simulink model "MSDR_DH_DeplV1sim"  (R2019a)
settings: Solver=ode45  StartTime=0.0  StopTime=simtime  FixedStep=0.1  MaxStep=ts_max  RelTol=rel_tolerance
values from neighbouring files (symbols this model uses):
  a_f = 1E-5*depl_fuel_temp_coef(depl_index)    [MSDR_DH_DeplV1para.m]
  a_g = 1E-5*depl_grap_temp_coef(depl_index)    [MSDR_DH_DeplV1para.m]
  A_s = 1.2245    [MSDR_DH_DeplV1para.m]
  beta = depl_beta(depl_index,:)    [MSDR_DH_DeplV1para.m]
  beta_t = sum(beta)    [MSDR_DH_DeplV1para.m]
  Cp_f = depl_Cp_Fuel_coef*1.355616e-3    [MSDR_DH_DeplV1para.m]
  Cp_p = Cp_s_shx    [MSDR_DH_DeplV1para.m]
  Cp_s = Cp_s*1e-6    (= 3.588208e-09)    [MSDR_DH_DeplV1para.m]
  Cp_sc = 4761.392e-6    (= 0.004761392)    [MSDR_DH_DeplV1para.m]
  Cp_w = 456.056e-6    (= 0.000456056)    [MSDR_DH_DeplV1para.m]
  D_it = 0.0141478    [MSDR_DH_DeplV1para.m]
  D_ot = 0.015875    [MSDR_DH_DeplV1para.m]
  DHRS_TIME_K = 10    [MSDR_DH_DeplV1para.m]
  dHs_dPs = -0.042433622114357    (= -0.0424336221144)    [MSDR_DH_DeplV1para.m]
  Epsilon = 1E-3    (= 0.001)    [MSDR_DH_DeplV1para.m]
  Fiss_factor = 2.464783802008740e-03    (= 0.00246478380201)    [MSDR_DH_DeplV1para.m]
  gamma0 = 9.635981959409105e-01    (= 0.963598195941)    [MSDR_DH_DeplV1para.m]
  gamma1 = 3.560674858154914e-02    (= 0.0356067485815)    [MSDR_DH_DeplV1para.m]
  gamma2 = 7.950554775404400e-04    (= 0.00079505547754)    [MSDR_DH_DeplV1para.m]
  gamma_I = 5.1135e-2    (= 0.051135)    [MSDR_DH_DeplV1para.m]
  gamma_Pm = 1.08E-2    (= 0.0108)    [MSDR_DH_DeplV1para.m]
  gamma_Xe = 1.1628e-2    (= 0.011628)    [MSDR_DH_DeplV1para.m]
  h_pw = h_s_shx    [MSDR_DH_DeplV1para.m]
  h_wb = 13349.334646671E-6    (= 0.0133493346467)    [MSDR_DH_DeplV1para.m]
  h_ws = 5732.378387768E-6    (= 0.00573237838777)    [MSDR_DH_DeplV1para.m]
  h_wsc = 8385.005556375E-6    (= 0.00838500555638)    [MSDR_DH_DeplV1para.m]
  hA_fg = [h_fg*A_fg/2, h_fg*A_fg/2]    [MSDR_DH_DeplV1para.m]
  hA_p_phx1 = h_p_phx*A_p_phx    [MSDR_DH_DeplV1para.m]
  hA_p_phx2 = h_p_phx*A_p_phx    [MSDR_DH_DeplV1para.m]
  hA_p_phx3 = h_p_phx*A_p_phx    [MSDR_DH_DeplV1para.m]
  hA_p_phx4 = h_p_phx*A_p_phx    [MSDR_DH_DeplV1para.m]
  hA_p_phx5 = h_p_phx*A_p_phx    [MSDR_DH_DeplV1para.m]
  hA_p_phx6 = h_p_phx*A_p_phx    [MSDR_DH_DeplV1para.m]
  hA_p_shx1 = h_p_shx*A_p_shx    [MSDR_DH_DeplV1para.m]
  hA_p_shx2 = h_p_shx*A_p_shx    [MSDR_DH_DeplV1para.m]
  hA_p_shx3 = h_p_shx*A_p_shx    [MSDR_DH_DeplV1para.m]
  hA_p_shx4 = h_p_shx*A_p_shx    [MSDR_DH_DeplV1para.m]
  hA_p_shx5 = h_p_shx*A_p_shx    [MSDR_DH_DeplV1para.m]
  hA_p_shx6 = h_p_shx*A_p_shx    [MSDR_DH_DeplV1para.m]
  hA_s_phx1 = h_s_phx*A_s_phx    [MSDR_DH_DeplV1para.m]
  hA_s_phx2 = h_s_phx*A_s_phx    [MSDR_DH_DeplV1para.m]
  hA_s_phx3 = h_s_phx*A_s_phx    [MSDR_DH_DeplV1para.m]
  hA_s_phx4 = h_s_phx*A_s_phx    [MSDR_DH_DeplV1para.m]
  hA_s_phx5 = h_s_phx*A_s_phx    [MSDR_DH_DeplV1para.m]
  hA_s_phx6 = h_s_phx*A_s_phx    [MSDR_DH_DeplV1para.m]
  hA_s_shx1 = h_s_shx*A_s_shx    [MSDR_DH_DeplV1para.m]
  hA_s_shx2 = h_s_shx*A_s_shx    [MSDR_DH_DeplV1para.m]
  hA_s_shx3 = h_s_shx*A_s_shx    [MSDR_DH_DeplV1para.m]
  hA_s_shx4 = h_s_shx*A_s_shx    [MSDR_DH_DeplV1para.m]
  hA_s_shx5 = h_s_shx*A_s_shx    [MSDR_DH_DeplV1para.m]
  hA_s_shx6 = h_s_shx*A_s_shx    [MSDR_DH_DeplV1para.m]
  I_0 = gamma_I*Sig_f_msdr*phi_0/lam_I    [MSDR_DH_DeplV1para.m]
  Ifa = [0.25, 0.25]    [MSDR_DH_DeplV1para.m]
  Ifb = [0.25, 0.25]    [MSDR_DH_DeplV1para.m]
  Ig = [0.5, 0.5]    [MSDR_DH_DeplV1para.m]
  K_1 = 11.632248097704855    (= 11.6322480977)    [MSDR_DH_DeplV1para.m]
  K_4 = b(1)    [MSDR_DH_DeplV1para.m]
  K_5 = a(1)    [MSDR_DH_DeplV1para.m]
  K_b = 12.834854076292217    (= 12.8348540763)    [MSDR_DH_DeplV1para.m]
  K_pump = 1/5    (= 0.2)    [MSDR_DH_DeplV1para.m]
  K_sc = -17.615718797133468    (= -17.6157187971)    [MSDR_DH_DeplV1para.m]
  ka = [0.235, 0.235]    [MSDR_DH_DeplV1para.m]
  kb = [0.235, 0.235]    [MSDR_DH_DeplV1para.m]
  kga = [0.015, 0.015]    [MSDR_DH_DeplV1para.m]
  kgb = [0.015, 0.015]    [MSDR_DH_DeplV1para.m]
  L = 8.5344    [MSDR_DH_DeplV1para.m]
  L_b = 2.3645    [MSDR_DH_DeplV1para.m]
  L_s = 4.723    [MSDR_DH_DeplV1para.m]
  Lam = depl_Lam(depl_index)    [MSDR_DH_DeplV1para.m]
  lam = [1.240E-02, 3.05E-02, 1.11E-01, 3.01E-01, 1.140E+00, 3.014E+00]    [MSDR_DH_DeplV1para.m]
  lam_bubl = 2.0e-2    (= 0.02)    [MSDR_DH_DeplV1para.m]
  lam_I = 2.875e-5    (= 2.875e-05)    [MSDR_DH_DeplV1para.m]
  lam_Pm = log(2)/(2.21*24*3600)    [MSDR_DH_DeplV1para.m]
  lam_Xe = 2.0916e-5    (= 2.0916e-05)    [MSDR_DH_DeplV1para.m]
  lambda0 = 0.0945298    [MSDR_DH_DeplV1para.m]
  lambda1 = 0.00441957    [MSDR_DH_DeplV1para.m]
  lambda2 = 8.60979e-05    [MSDR_DH_DeplV1para.m]
  m_3m = W_3*2    (= 8618.207327)    [MSDR_DH_DeplV1para.m]
  m_f_t = total_mp_phx + core_fm + mp_phxm*3 + m_fm    [MSDR_DH_DeplV1para.m]
  m_fm = W_f*1    (= 4989.48)    [MSDR_DH_DeplV1para.m]
  M_stm = 0.018    [MSDR_DH_DeplV1para.m]
  mcp_fa = mfa*Cp_f    [MSDR_DH_DeplV1para.m]
  mcp_fb = mfb*Cp_f    [MSDR_DH_DeplV1para.m]
  mcp_g = mg*Cp_g    [MSDR_DH_DeplV1para.m]
  mcp_p_phx1 = Cp_p_phx*mp_phx1    [MSDR_DH_DeplV1para.m]
  mcp_p_phx2 = Cp_p_phx*mp_phx2    [MSDR_DH_DeplV1para.m]
  mcp_p_phx3 = Cp_p_phx*mp_phx3    [MSDR_DH_DeplV1para.m]
  mcp_p_phx4 = Cp_p_phx*mp_phx4    [MSDR_DH_DeplV1para.m]
  mcp_p_phx5 = Cp_p_phx*mp_phx5    [MSDR_DH_DeplV1para.m]
  mcp_p_phx6 = Cp_p_phx*mp_phx6    [MSDR_DH_DeplV1para.m]
  mcp_p_shx1 = Cp_p_shx*mp_shx1    [MSDR_DH_DeplV1para.m]
  mcp_p_shx2 = Cp_p_shx*mp_shx2    [MSDR_DH_DeplV1para.m]
  mcp_p_shx3 = Cp_p_shx*mp_shx3    [MSDR_DH_DeplV1para.m]
  mcp_p_shx4 = Cp_p_shx*mp_shx4    [MSDR_DH_DeplV1para.m]
  mcp_p_shx5 = Cp_p_shx*mp_shx5    [MSDR_DH_DeplV1para.m]
  mcp_p_shx6 = Cp_p_shx*mp_shx6    [MSDR_DH_DeplV1para.m]
  mcp_s_phx1 = Cp_s_phx*ms_phx1    [MSDR_DH_DeplV1para.m]
  mcp_s_phx2 = Cp_s_phx*ms_phx2    [MSDR_DH_DeplV1para.m]
  mcp_s_phx3 = Cp_s_phx*ms_phx3    [MSDR_DH_DeplV1para.m]
  mcp_s_phx4 = Cp_s_phx*ms_phx4    [MSDR_DH_DeplV1para.m]
  mcp_s_phx5 = Cp_s_phx*ms_phx5    [MSDR_DH_DeplV1para.m]
  mcp_s_phx6 = Cp_s_phx*ms_phx6    [MSDR_DH_DeplV1para.m]
  mcp_s_shx1 = Cp_s_shx*ms_shx1    [MSDR_DH_DeplV1para.m]
  mcp_s_shx2 = Cp_s_shx*ms_shx1    [MSDR_DH_DeplV1para.m]
  mcp_s_shx3 = Cp_s_shx*ms_shx1    [MSDR_DH_DeplV1para.m]
  mcp_s_shx4 = Cp_s_shx*ms_shx1    [MSDR_DH_DeplV1para.m]
  mcp_s_shx5 = Cp_s_shx*ms_shx1    [MSDR_DH_DeplV1para.m]
  mcp_s_shx6 = Cp_s_shx*ms_shx1    [MSDR_DH_DeplV1para.m]
  mcp_t_phx1 = Cp_t_phx*mt_phx1    [MSDR_DH_DeplV1para.m]
  mcp_t_phx2 = Cp_t_phx*mt_phx2    [MSDR_DH_DeplV1para.m]
  mcp_t_phx3 = Cp_t_phx*mt_phx3    [MSDR_DH_DeplV1para.m]
  mcp_t_phx4 = Cp_t_phx*mt_phx4    [MSDR_DH_DeplV1para.m]
  mcp_t_phx5 = Cp_t_phx*mt_phx5    [MSDR_DH_DeplV1para.m]
  mcp_t_phx6 = Cp_t_phx*mt_phx6    [MSDR_DH_DeplV1para.m]
  mcp_t_shx1 = Cp_t_phx*mt_shx1    [MSDR_DH_DeplV1para.m]
  mcp_t_shx2 = Cp_t_phx*mt_shx2    [MSDR_DH_DeplV1para.m]
  mcp_t_shx3 = Cp_t_phx*mt_shx3    [MSDR_DH_DeplV1para.m]
  mcp_t_shx4 = Cp_t_phx*mt_shx4    [MSDR_DH_DeplV1para.m]
  mcp_t_shx5 = Cp_t_phx*mt_shx5    [MSDR_DH_DeplV1para.m]
  mcp_t_shx6 = Cp_t_phx*mt_shx6    [MSDR_DH_DeplV1para.m]
  ... (+159 more)
undefined symbols (not defined in the file or in its folder): C0, DHRS_MODE, DHRS_Power, DHRS_time, ln, P, Trip_P1_pump, Trip_P2_pump, Trip_P3_pump, Trip_S1_pump, Trip_S2_pump, Trip_S3_pump, Trip_T1_pump, Trip_T2_pump, Trip_T3_pump, Trip_UHX
libraries: simulink x2
(part 1 of 4)
settings Model: Creator=viikr  LastModifiedBy=visura
settings SolverCC: SolverJacobianMethodControl=FullAnalytical  AlgebraicLoopSolver=LineSearch
settings DataIOCC: ReturnWorkspaceOutputs=off
settings DebuggingCC: PregeneratedLibrarySubsystemCodeDiagnostic=none  ArithmeticOperatorsInVariantConditions=warning
settings SFSimCC: SimUseLocalCustomCode=off
settings RTWCC: RTWUseLocalCustomCode=off

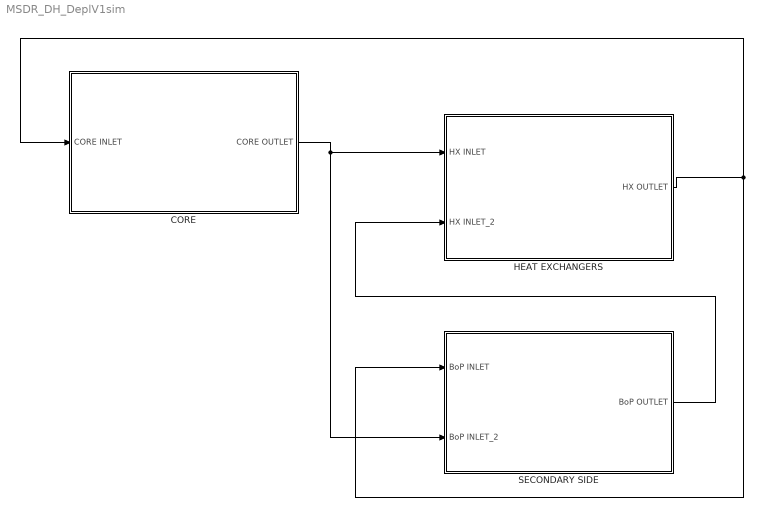
== system MSDR_DH_DeplV1sim ==
  CORE : Subsystem
  HEAT EXCHANGERS : Subsystem
  SECONDARY SIDE : Subsystem
  wires:
  SECONDARY SIDE/1(BoP OUTLET) -> HEAT EXCHANGERS/2(HX INLET_2)
  HEAT EXCHANGERS/1(HX OUTLET) -> SECONDARY SIDE/1(BoP INLET), CORE/1(CORE INLET)
  CORE/1(CORE OUTLET) -> SECONDARY SIDE/2(BoP INLET_2), HEAT EXCHANGERS/1(HX INLET)

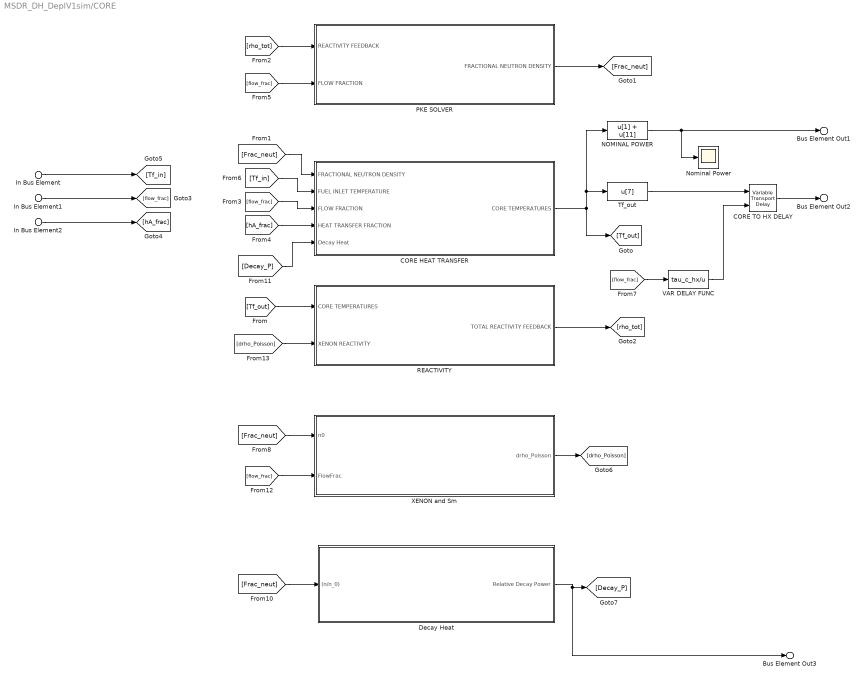
== system MSDR_DH_DeplV1sim/CORE ==
  In Bus Element2 : Inport  PortName=CORE INLET  Element=FUEL HEAT TRANSFER FRACTION
  In Bus Element : Inport  PortName=CORE INLET  Element=HX FUEL OUTLET TEMPERATURE
  In Bus Element1 : Inport  PortName=CORE INLET  Element=FUEL FLOW FRACTION
  CORE HEAT TRANSFER : Subsystem
  CORE TO HX DELAY : VariableTransportDelay  MaximumDelay=10000000  InitialOutput=T0_fb(2)
  Decay Heat : Subsystem
  NOMINAL POWER : Fcn  Expr=u[1] + u[11]
  Nominal Power : Scope
  PKE SOLVER : Subsystem
  REACTIVITY : Subsystem
  Tf_out : Fcn  Expr=u[7]
  VAR DELAY FUNC : Fcn  Expr=tau_c_hx/u
  XENON and Sm : Subsystem
  Bus Element Out2 : Outport  PortName=CORE OUTLET  Element=CORE FUEL OUTLET TEMPERATURE
  Bus Element Out1 : Outport  PortName=CORE OUTLET  Element=CORE POWER
  Bus Element Out3 : Outport  PortName=CORE OUTLET  Element=DECAY HEAT
  wires:
  Tf_out/1 -> CORE TO HX DELAY/1
  CORE HEAT TRANSFER/1(CORE TEMPERATURES) -> Tf_out/1, NOMINAL POWER/1, [Tf_out]
  [Tf_out] -> REACTIVITY/1(CORE TEMPERATURES)
  PKE SOLVER/1(FRACTIONAL NEUTRON DENSITY) -> [Frac_neut]
  [Frac_neut] -> CORE HEAT TRANSFER/1(FRACTIONAL NEUTRON DENSITY)
  REACTIVITY/1(TOTAL REACTIVITY FEEDBACK) -> [rho_tot]
  [flow_frac] -> PKE SOLVER/2(FLOW FRACTION)
  [flow_frac] -> CORE HEAT TRANSFER/3(FLOW FRACTION)
  [hA_frac] -> CORE HEAT TRANSFER/4(HEAT TRANSFER FRACTION)
  CORE TO HX DELAY/1 -> Bus Element Out2/1
  [flow_frac] -> VAR DELAY FUNC/1
  VAR DELAY FUNC/1 -> CORE TO HX DELAY/2
  [Tf_in] -> CORE HEAT TRANSFER/2(FUEL INLET TEMPERATURE)
  XENON and Sm/1(drho_Poisson) -> [drho_Poisson]
  [Frac_neut] -> XENON and Sm/1(n0)
  In Bus Element1/1 -> [flow_frac]
  In Bus Element2/1 -> [hA_frac]
  In Bus Element/1 -> [Tf_in]
  [drho_Poisson] -> REACTIVITY/2(XENON REACTIVITY)
  [rho_tot] -> PKE SOLVER/1(REACTIVITY FEEDBACK)
  [Frac_neut] -> Decay Heat/1((n/n_0))
  Decay Heat/1("Relative Decay Power ") -> Bus Element Out3/1, [Decay_P]
  [Decay_P] -> CORE HEAT TRANSFER/5(Decay Heat)
  NOMINAL POWER/1 -> Nominal Power/1, Bus Element Out1/1
  [flow_frac] -> XENON and Sm/2(FlowFrac)

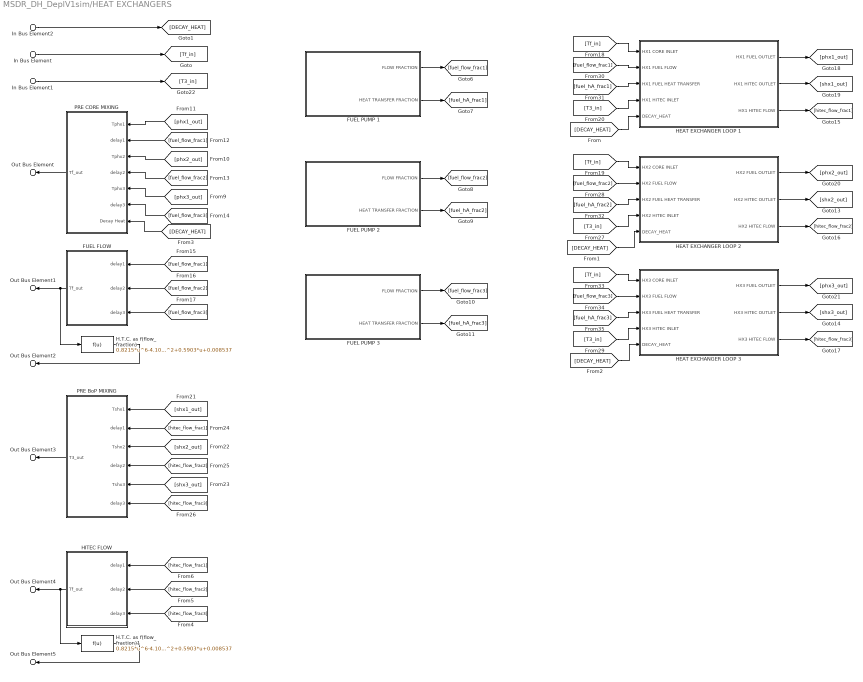
== system MSDR_DH_DeplV1sim/HEAT EXCHANGERS ==
  In Bus Element : Inport  PortName=HX INLET  Element=CORE FUEL OUTLET TEMPERATURE
  In Bus Element2 : Inport  PortName=HX INLET  Element=DECAY HEAT
  In Bus Element1 : Inport  Port=2  PortName=HX INLET_2  Element=BoP HITEC OUTLET TEMPERATURE
  FUEL FLOW : Subsystem
  FUEL PUMP 1 : Subsystem
  FUEL PUMP 2 : Subsystem
  FUEL PUMP 3 : Subsystem
  H.T.C. as f(flow_fraction) : Fcn  Expr=0.8215*u^6-4.108*u^5+7.848*u^4-7.165*u^3+3.004*u^2+0.5903*u+0.008537
  H.T.C. as f(flow_fraction)1 : Fcn  Expr=0.8215*u^6-4.108*u^5+7.848*u^4-7.165*u^3+3.004*u^2+0.5903*u+0.008537
  HEAT EXCHANGER LOOP 1 : Subsystem
  HEAT EXCHANGER LOOP 2 : Subsystem
  HEAT EXCHANGER LOOP 3 : Subsystem
  HITEC FLOW : Subsystem
  PRE BoP MIXING : Subsystem
  PRE CORE MIXING : Subsystem
  Out Bus Element : Outport  PortName=HX OUTLET  Element=HX FUEL OUTLET TEMPERATURE
  Out Bus Element1 : Outport  PortName=HX OUTLET  Element=FUEL FLOW FRACTION
  Out Bus Element2 : Outport  PortName=HX OUTLET  Element=FUEL HEAT TRANSFER FRACTION
  Out Bus Element3 : Outport  PortName=HX OUTLET  Element=HX HITEC OUTLET TEMPERATURE
  Out Bus Element4 : Outport  PortName=HX OUTLET  Element=HITEC FLOW FRACTION
  Out Bus Element5 : Outport  PortName=HX OUTLET  Element=HITEC HEAT TRANSFER FRACTION
  wires:
  In Bus Element/1 -> [Tf_in]
  FUEL PUMP 1/1(FLOW FRACTION) -> [fuel_flow_frac1]
  FUEL PUMP 1/2(HEAT TRANSFER FRACTION) -> [fuel_hA_frac1]
  FUEL PUMP 2/2(HEAT TRANSFER FRACTION) -> [fuel_hA_frac2]
  FUEL PUMP 2/1(FLOW FRACTION) -> [fuel_flow_frac2]
  FUEL PUMP 3/2(HEAT TRANSFER FRACTION) -> [fuel_hA_frac3]
  FUEL PUMP 3/1(FLOW FRACTION) -> [fuel_flow_frac3]
  [phx1_out] -> PRE CORE MIXING/1(Tphx1)
  [fuel_flow_frac1] -> PRE CORE MIXING/2(delay1)
  [phx2_out] -> PRE CORE MIXING/3(Tphx2)
  [fuel_flow_frac2] -> PRE CORE MIXING/4(delay2)
  [phx3_out] -> PRE CORE MIXING/5(Tphx3)
  [fuel_flow_frac3] -> PRE CORE MIXING/6(delay3)
  PRE CORE MIXING/1(Tf_out) -> Out Bus Element/1
  FUEL FLOW/1(Tf_out) -> H.T.C. as f(flow_fraction)/1, Out Bus Element1/1
  H.T.C. as f(flow_fraction)/1 -> Out Bus Element2/1
  [hitec_flow_frac2] -> PRE BoP MIXING/4(delay2)
  [hitec_flow_frac1] -> PRE BoP MIXING/2(delay1)
  [shx2_out] -> PRE BoP MIXING/3(Tshx2)
  [shx3_out] -> PRE BoP MIXING/5(Tshx3)
  [hitec_flow_frac3] -> PRE BoP MIXING/6(delay3)
  [shx1_out] -> PRE BoP MIXING/1(Tshx1)
  PRE BoP MIXING/1(T3_out) -> Out Bus Element3/1
  HEAT EXCHANGER LOOP 2/2(HX2 HITEC OUTLET) -> [shx2_out]
  [T3_in] -> HEAT EXCHANGER LOOP 3/4(HX3 HITEC INLET)
  HEAT EXCHANGER LOOP 3/3(HX3 HITEC FLOW) -> [hitec_flow_frac3]
  HEAT EXCHANGER LOOP 2/3(HX2 HITEC FLOW) -> [hitec_flow_frac2]
  HEAT EXCHANGER LOOP 1/3(HX1 HITEC FLOW) -> [hitec_flow_frac1]
  HEAT EXCHANGER LOOP 3/2(HX3 HITEC OUTLET) -> [shx3_out]
  HEAT EXCHANGER LOOP 1/2(HX1 HITEC OUTLET) -> [shx1_out]
  [T3_in] -> HEAT EXCHANGER LOOP 1/4(HX1 HITEC INLET)
  HEAT EXCHANGER LOOP 1/1(HX1 FUEL OUTLET) -> [phx1_out]
  [fuel_flow_frac3] -> HEAT EXCHANGER LOOP 3/2(HX3 FUEL FLOW)
  [Tf_in] -> HEAT EXCHANGER LOOP 2/1(HX2 CORE INLET)
  [T3_in] -> HEAT EXCHANGER LOOP 2/4(HX2 HITEC INLET)
  [fuel_hA_frac2] -> HEAT EXCHANGER LOOP 2/3(HX2 FUEL HEAT TRANSFER)
  [fuel_flow_frac2] -> HEAT EXCHANGER LOOP 2/2(HX2 FUEL FLOW)
  [Tf_in] -> HEAT EXCHANGER LOOP 3/1(HX3 CORE INLET)
  [fuel_hA_frac1] -> HEAT EXCHANGER LOOP 1/3(HX1 FUEL HEAT TRANSFER)
  [Tf_in] -> HEAT EXCHANGER LOOP 1/1(HX1 CORE INLET)
  [fuel_hA_frac3] -> HEAT EXCHANGER LOOP 3/3(HX3 FUEL HEAT TRANSFER)
  HEAT EXCHANGER LOOP 3/1(HX3 FUEL OUTLET) -> [phx3_out]
  HEAT EXCHANGER LOOP 2/1(HX2 FUEL OUTLET) -> [phx2_out]
  In Bus Element1/1 -> [T3_in]
  [fuel_flow_frac1] -> HEAT EXCHANGER LOOP 1/2(HX1 FUEL FLOW)
  [fuel_flow_frac1] -> FUEL FLOW/1(delay1)
  [fuel_flow_frac2] -> FUEL FLOW/2(delay2)
  [fuel_flow_frac3] -> FUEL FLOW/3(delay3)
  In Bus Element2/1 -> [DECAY_HEAT]
  [DECAY_HEAT] -> HEAT EXCHANGER LOOP 1/5(DECAY_HEAT)
  [DECAY_HEAT] -> HEAT EXCHANGER LOOP 2/5(DECAY_HEAT)
  [DECAY_HEAT] -> HEAT EXCHANGER LOOP 3/5(DECAY_HEAT)
  [DECAY_HEAT] -> PRE CORE MIXING/7(Decay Heat)
  [hitec_flow_frac1] -> HITEC FLOW/1(delay1)
  [hitec_flow_frac2] -> HITEC FLOW/2(delay2)
  [hitec_flow_frac3] -> HITEC FLOW/3(delay3)
  HITEC FLOW/1(Tf_out) -> H.T.C. as f(flow_fraction)1/1, Out Bus Element4/1
  H.T.C. as f(flow_fraction)1/1 -> Out Bus Element5/1

== system MSDR_DH_DeplV1sim/SECONDARY SIDE ==
  In Bus Element : Inport  PortName=BoP INLET  Element=HX HITEC OUTLET TEMPERATURE
  In Bus Element2 : Inport  PortName=BoP INLET  Element=HITEC FLOW FRACTION
  In Bus Element3 : Inport  PortName=BoP INLET  Element=HITEC HEAT TRANSFER FRACTION
  In Bus Element1 : Inport  Port=2  PortName=BoP INLET_2  Element=CORE POWER
  OTSG + BALANCE OF PLANT : Subsystem  Commented=on
  Variant Subsystem : Subsystem  Variant=on
  Bus Element Out2 : Outport  PortName=BoP OUTLET  Element=BoP HITEC OUTLET TEMPERATURE
  wires:
  Variant Subsystem/1(HITEC_OUTLET) -> Bus Element Out2/1
  In Bus Element3/1 -> Variant Subsystem/4(HITEC_HTC_FRAC)
  In Bus Element2/1 -> Variant Subsystem/3(HITEC_FLOW_FRAC)
  In Bus Element/1 -> Variant Subsystem/1(HITEC_INLET)
  In Bus Element1/1 -> Variant Subsystem/2(POWER LEVEL)

== system MSDR_DH_DeplV1sim/CORE/CORE HEAT TRANSFER ==
  FRACTIONAL NEUTRON DENSITY : Inport
  FUEL INLET TEMPERATURE : Inport  Port=2
  FLOW FRACTION : Inport  Port=3
  HEAT TRANSFER FRACTION : Inport  Port=4
  Decay Heat : Inport  Port=5
  Mux : Mux  Inputs=11
      settings: DisplayOption=signals
  T_f1a : Integrator  InitialCondition=T0_fa(1)
  T_f1b : Integrator  InitialCondition=T0_fb(1)
  T_f2a : Integrator  InitialCondition=T0_fa(2)
  T_f2b : Integrator  InitialCondition=T0_fb(2)
  T_g1 : Integrator  InitialCondition=T0_g(1)
  T_g2 : Integrator  InitialCondition=T0_g(2)
  To Workspace : ToWorkspace  VariableName=core_ht  SampleTime=-1
  d(T_f1a)/dt : Fcn  Expr=((u[9]*W_f/mfa(1))*(u[2] - u[3])) + (ka(1)*P*u[1]/mcp_fa(1)) + (kga(1)*u[10]*hA_fg(1)*(u[5] - u[3]))/((kga(1)+kgb(1))*mcp_fa(1)) + u(11)*P*mfa(1)/(m_f_t*mcp_fa(1))
  d(T_f1a)/dt1 : Fcn  Expr=(1-0.07)*u
  d(T_f1b)/dt : Fcn  Expr=((u[9]*W_f/mfb(1))*(u[3] - u[4])) + (kb(1)*P*u[1]/mcp_fb(1)) + (kgb(1)*u[10]*hA_fg(1)*(u[5] - u[3]))/((kga(1)+kgb(1))*mcp_fb(1)) + u(11)*P*mfb(1)/(m_f_t*mcp_fb(1))
  d(T_f2a)/dt : Fcn  Expr=((u[9]*W_f/mfa(2))*(u[4] - u[6])) + (ka(2)*P*u[1]/mcp_fa(2)) + (kga(2)*u[10]*hA_fg(2)*(u[8] - u[6]))/((kga(2)+kgb(2))*mcp_fa(2)) + u(11)*P*mfa(2)/(m_f_t*mcp_fa(2))
  d(T_f2b)/dt : Fcn  Expr=((u[9]*W_f/mfb(2))*(u[6] - u[7])) + (kb(2)*P*u[1]/mcp_fb(2)) + (kgb(2)*u[10]*hA_fg(2)*(u[8] - u[6]))/((kga(2)+kgb(2))*mcp_fb(2)) + u(11)*P*mfb(2)/(m_f_t*mcp_fb(2))
  d(T_g1)/dt : Fcn  Expr=(u[10]*hA_fg(1)/mcp_g(1))*(u[3] - u[5]) + (kga(1)+kgb(1))*P*u[1]/mcp_g(1)
  d(T_g2)/dt : Fcn  Expr=(u[10]*hA_fg(2)/mcp_g(2))*(u[6] - u[8]) + (kga(2)+kgb(2))*P*u[1]/mcp_g(2)
  CORE TEMPERATURES : Outport
  wires:
  d(T_f1b)/dt/1 -> T_f1b/1
  d(T_f1a)/dt/1 -> T_f1a/1
  d(T_g1)/dt/1 -> T_g1/1
  FUEL INLET TEMPERATURE/1 -> Mux/2
  T_f1a/1 -> Mux/3
  T_f1b/1 -> Mux/4
  T_g1/1 -> Mux/5
  d(T_f2a)/dt/1 -> T_f2a/1
  d(T_f2b)/dt/1 -> T_f2b/1
  T_g2/1 -> Mux/8
  d(T_g2)/dt/1 -> T_g2/1
  T_f2a/1 -> Mux/6
  T_f2b/1 -> Mux/7
  Mux/1 -> To Workspace/1, CORE TEMPERATURES/1, d(T_g2)/dt/1, d(T_f2b)/dt/1, d(T_f2a)/dt/1, d(T_g1)/dt/1, d(T_f1b)/dt/1, d(T_f1a)/dt/1
  FLOW FRACTION/1 -> Mux/9
  HEAT TRANSFER FRACTION/1 -> Mux/10
  Decay Heat/1 -> Mux/11
  d(T_f1a)/dt1/1 -> Mux/1
  FRACTIONAL NEUTRON DENSITY/1 -> d(T_f1a)/dt1/1

== system MSDR_DH_DeplV1sim/CORE/Decay Heat ==
  (n/n_0) : Inport
  Decay Power Percentage : Fcn  Expr=u(2)+u(3)+u(4)
  Decay Precursor G1 : Fcn  Expr=u(1)*Fiss_factor*gamma0 - lambda0*u(2)
  Decay Precursor G2 : Fcn  Expr=u(1)*Fiss_factor*gamma1 - lambda1*u(3)
  Decay Precursor G3 : Fcn  Expr=u(1)*Fiss_factor*gamma2 - lambda2*u(4)
  Integrator : Integrator  InitialCondition=0.025125
  Integrator1 : Integrator  InitialCondition=0.0198578
  Integrator2 : Integrator  InitialCondition=0.0227606
  Mux : Mux
      settings: DisplayOption=signals
  Scope : Scope
  To Workspace : ToWorkspace  VariableName=Decay_Group_total  SampleTime=-1
  To Workspace1 : ToWorkspace  VariableName=Decay_Groups1  SampleTime=-1
  To Workspace2 : ToWorkspace  VariableName=Decay_Groups2  SampleTime=-1
  To Workspace3 : ToWorkspace  VariableName=Decay_Groups3  SampleTime=-1
  "Relative Decay Power " : Outport
  wires:
  Decay Power Percentage/1 -> "Relative Decay Power "/1, Scope/1, To Workspace/1
  Decay Precursor G1/1 -> Integrator/1
  Decay Precursor G2/1 -> Integrator1/1
  Decay Precursor G3/1 -> Integrator2/1
  Mux/1 -> Decay Precursor G3/1, Decay Precursor G2/1, Decay Precursor G1/1, Decay Power Percentage/1
  Integrator/1 -> Mux/2, To Workspace1/1
  Integrator1/1 -> Mux/3, To Workspace2/1
  Integrator2/1 -> Mux/4, To Workspace3/1
  (n/n_0)/1 -> Mux/1

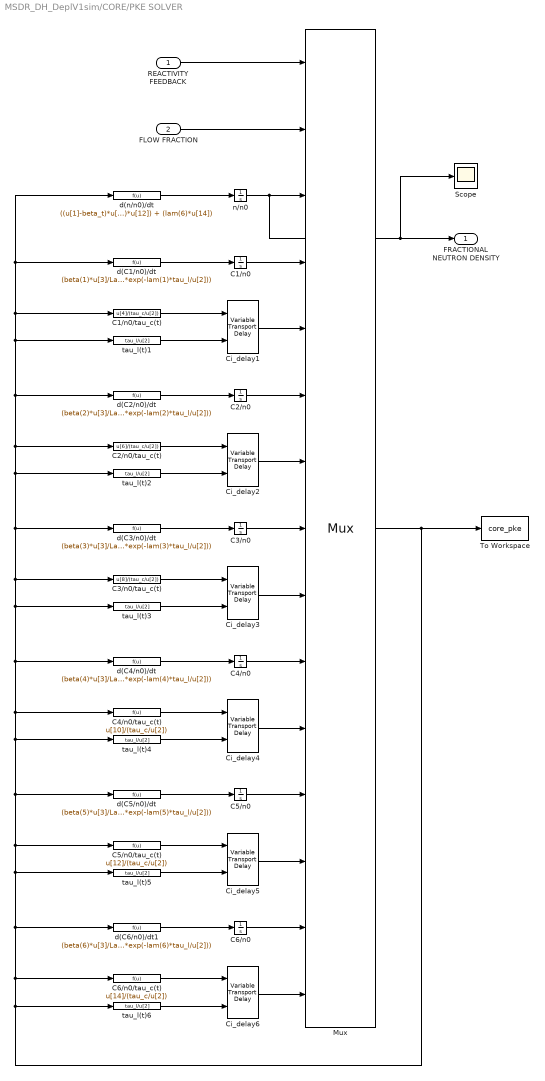
== system MSDR_DH_DeplV1sim/CORE/PKE SOLVER ==
  REACTIVITY FEEDBACK : Inport
  FLOW FRACTION : Inport  Port=2
  C1/n0 : Integrator  InitialCondition=C0(1)
  C1/n0/tau_c(t) : Fcn  Expr=u[4]/(tau_c/u[2])
  C2/n0 : Integrator  InitialCondition=C0(2)
  C2/n0/tau_c(t) : Fcn  Expr=u[6]/(tau_c/u[2])
  C3/n0 : Integrator  InitialCondition=C0(3)
  C3/n0/tau_c(t) : Fcn  Expr=u[8]/(tau_c/u[2])
  C4/n0 : Integrator  InitialCondition=C0(4)
  C4/n0/tau_c(t) : Fcn  Expr=u[10]/(tau_c/u[2])
  C5/n0 : Integrator  InitialCondition=C0(5)
  C5/n0/tau_c(t) : Fcn  Expr=u[12]/(tau_c/u[2])
  C6/n0 : Integrator  InitialCondition=C0(6)
  C6/n0/tau_c(t) : Fcn  Expr=u[14]/(tau_c/u[2])
  Ci_delay1 : VariableTransportDelay  MaximumDelay=1000000  InitialOutput=C0(1)/tau_c
  Ci_delay2 : VariableTransportDelay  MaximumDelay=1000000  InitialOutput=C0(2)/tau_c
  Ci_delay3 : VariableTransportDelay  MaximumDelay=1000000  InitialOutput=C0(3)/tau_c
  Ci_delay4 : VariableTransportDelay  MaximumDelay=1000000  InitialOutput=C0(4)/tau_c
  Ci_delay5 : VariableTransportDelay  MaximumDelay=1000000  InitialOutput=C0(5)/tau_c
  Ci_delay6 : VariableTransportDelay  MaximumDelay=1000000  InitialOutput=C0(6)/tau_c
  Mux : Mux  Inputs=15
      settings: DisplayOption=signals
  Scope : Scope
  To Workspace : ToWorkspace  VariableName=core_pke  SampleTime=-1
  d(C1/n0)/dt : Fcn  Expr=(beta(1)*u[3]/Lam) - (lam(1)*u[4]) - (u[4]/(tau_c/u[2])) + (u[5]*exp(-lam(1)*tau_l/u[2]))
  d(C2/n0)/dt : Fcn  Expr=(beta(2)*u[3]/Lam) - (lam(2)*u[6]) - (u[6]/(tau_c/u[2])) + (u[7]*exp(-lam(2)*tau_l/u[2]))
  d(C3/n0)/dt : Fcn  Expr=(beta(3)*u[3]/Lam) - (lam(3)*u[8]) - (u[8]/(tau_c/u[2])) + (u[9]*exp(-lam(3)*tau_l/u[2]))
  d(C4/n0)/dt : Fcn  Expr=(beta(4)*u[3]/Lam) - (lam(4)*u[10]) - (u[10]/(tau_c/u[2])) + (u[11]*exp(-lam(4)*tau_l/u[2]))
  d(C5/n0)/dt : Fcn  Expr=(beta(5)*u[3]/Lam) - (lam(5)*u[12]) - (u[12]/(tau_c/u[2])) + (u[13]*exp(-lam(5)*tau_l/u[2]))
  d(C6/n0)/dt1 : Fcn  Expr=(beta(6)*u[3]/Lam) - (lam(6)*u[14]) - (u[14]/(tau_c/u[2])) + (u[14]*exp(-lam(6)*tau_l/u[2]))
  d(n/n0)/dt : Fcn  Expr=((u[1]-beta_t)*u[3]/Lam) + (lam(1)*u[4]) + (lam(2)*u[6]) + (lam(3)*u[8]) + (lam(4)*u[10]) + (lam(5)*u[12]) + (lam(6)*u[14])
  n/n0 : Integrator  InitialCondition=n0
  tau_l(t){1..6} (6 alike) : Fcn  Expr=tau_l/u[2]
  FRACTIONAL NEUTRON DENSITY : Outport
  wires:
  C1/n0/tau_c(t)/1 -> Ci_delay1/1
  d(n/n0)/dt/1 -> n/n0/1
  d(C1/n0)/dt/1 -> C1/n0/1
  REACTIVITY FEEDBACK/1 -> Mux/1
  n/n0/1 -> Scope/1, FRACTIONAL NEUTRON DENSITY/1, Mux/3
  FLOW FRACTION/1 -> Mux/2
  C1/n0/1 -> Mux/4
  Ci_delay1/1 -> Mux/5
  tau_l(t)1/1 -> Ci_delay1/2
  C2/n0/tau_c(t)/1 -> Ci_delay2/1
  d(C2/n0)/dt/1 -> C2/n0/1
  tau_l(t)2/1 -> Ci_delay2/2
  Ci_delay2/1 -> Mux/7
  C2/n0/1 -> Mux/6
  C3/n0/1 -> Mux/8
  d(C3/n0)/dt/1 -> C3/n0/1
  tau_l(t)3/1 -> Ci_delay3/2
  Ci_delay3/1 -> Mux/9
  C3/n0/tau_c(t)/1 -> Ci_delay3/1
  C4/n0/1 -> Mux/10
  C4/n0/tau_c(t)/1 -> Ci_delay4/1
  tau_l(t)4/1 -> Ci_delay4/2
  d(C4/n0)/dt/1 -> C4/n0/1
  Ci_delay4/1 -> Mux/11
  C5/n0/tau_c(t)/1 -> Ci_delay5/1
  d(C5/n0)/dt/1 -> C5/n0/1
  tau_l(t)5/1 -> Ci_delay5/2
  C5/n0/1 -> Mux/12
  Ci_delay5/1 -> Mux/13
  C6/n0/1 -> Mux/14
  tau_l(t)6/1 -> Ci_delay6/2
  d(C6/n0)/dt1/1 -> C6/n0/1
  C6/n0/tau_c(t)/1 -> Ci_delay6/1
  Ci_delay6/1 -> Mux/15
  Mux/1 -> To Workspace/1, tau_l(t)6/1, d(n/n0)/dt/1, d(C1/n0)/dt/1, C1/n0/tau_c(t)/1, tau_l(t)1/1, d(C2/n0)/dt/1, C2/n0/tau_c(t)/1, tau_l(t)2/1, d(C3/n0)/dt/1, C3/n0/tau_c(t)/1, tau_l(t)3/1, d(C4/n0)/dt/1, C4/n0/tau_c(t)/1, tau_l(t)4/1, d(C5/n0)/dt/1, C5/n0/tau_c(t)/1, tau_l(t)5/1, d(C6/n0)/dt1/1, C6/n0/tau_c(t)/1

== system MSDR_DH_DeplV1sim/CORE/REACTIVITY ==
  CORE TEMPERATURES : Inport
  XENON REACTIVITY : Inport  Port=2
  From Workspace : FromWorkspace  VariableName=react  SampleTime=1  Interpolate=off  OutputAfterFinalValue=Holding final value
  Sum1 : Sum
  Sum2 : Sum  Inputs=++++
  To Workspace : ToWorkspace  VariableName=core_react  SampleTime=-1
  To Workspace1 : ToWorkspace  VariableName=rho_fb_f  SampleTime=-1
  To Workspace2 : ToWorkspace  VariableName=rho_fb_g  SampleTime=-1
  To Workspace3 : ToWorkspace  VariableName=rho_fb_tot  SampleTime=-1
  dkf : Fcn  Expr=Ifa(1)*(u[3]-T0_fa(1)) + Ifb(1)*(u[4]-T0_fb(1)) + Ifa(2)*(u[6]-T0_fa(2)) + Ifb(2)*(u[7]-T0_fb(2))
  dkg : Fcn  Expr=Ig(1)*(u[5]-T0_g(1)) + Ig(2)*(u[8]-T0_g(2))
  fuel : Gain  Gain=a_f
  graphite : Gain  Gain=a_g
  rho_0 : Constant  Value=rho_0
  TOTAL REACTIVITY FEEDBACK : Outport
  wires:
  graphite/1 -> To Workspace2/1, Sum1/2
  fuel/1 -> Sum1/1, To Workspace1/1
  dkg/1 -> graphite/1
  dkf/1 -> fuel/1
  CORE TEMPERATURES/1 -> dkf/1, dkg/1
  Sum1/1 -> To Workspace3/1, Sum2/2
  XENON REACTIVITY/1 -> Sum2/1
  Sum2/1 -> To Workspace/1, TOTAL REACTIVITY FEEDBACK/1
  rho_0/1 -> Sum2/3
  From Workspace/1 -> Sum2/4

== system MSDR_DH_DeplV1sim/CORE/XENON and Sm ==
  n0 : Inport
  FlowFrac : Inport  Port=2
  Add : Sum
  Integrator1 : Integrator  InitialCondition=Xe_0
  Integrator2 : Integrator  InitialCondition=Xe_og
  Integrator3 : Integrator  InitialCondition=Pm_0
  Integrator30 : Integrator  InitialCondition=I_0
  Integrator4 : Integrator  InitialCondition=Sm_0
  Mux : Mux  Inputs=5
      settings: DisplayOption=signals
  Mux1 : Mux  Inputs=7
      settings: DisplayOption=signals
  To Workspace : ToWorkspace  VariableName=msbr_poisons  SampleTime=-1
  To Workspace1 : ToWorkspace  VariableName=msbr_poisons_Sm  SampleTime=-1
  Unit Delay : UnitDelay  SampleTime=-1  HasFrameUpgradeWarning=on
  Unit Delay1 : UnitDelay  InitialCondition=tau_c  SampleTime=-1  HasFrameUpgradeWarning=on
  Unit Delay2 : UnitDelay  InitialCondition=Sm_0_core  SampleTime=-1  HasFrameUpgradeWarning=on
  Unit Delay3 : UnitDelay  SampleTime=-1  HasFrameUpgradeWarning=on
  d(I(t)/I0)/dt : Fcn  Expr=(gamma_I*Sig_f_msdr*phi_0)*u[1] - lam_I*u[2]
  d(Pm(t))/dt : Fcn  Expr=gamma_Pm*Sig_f_msdr*phi_0*u[1] - lam_Pm*u[4]
  d(Sm(t))/dt : Fcn  Expr=lam_Pm*u[4] - sig_Sm*u[6]*phi_0*u[1]
  d(Sm_core(t))/dt : Fcn  Expr=u[5]*(u[3]/((tau_c+tau_l)/u[2]))
  d(Xe(t)/X0)/dt : Fcn  Expr=(gamma_Xe*Sig_f_msdr*phi_0)*u[1] + lam_I*u[2] - lam_Xe*u[3] - sig_Xe*phi_0*u[1]*u[3] - lam_bubl*u[3]
  d(Xe_og(t)/X0_og)/dt1 : Fcn  Expr=lam_bubl*u[3] - lam_Xe*u[4]
  drho_Sm_core : Fcn  Expr=-rhoSm_0*((u[6]/Sm_0_core)-1)
  drho_poison : Fcn  Expr=rhoXe_0*((u[3]/Xe_0)-1)
  tau_c(t) : Fcn  Expr=tau_c/u[2]
  drho_Poisson : Outport
  wires:
  Integrator1/1 -> Mux/3
  Mux/1 -> d(Xe_og(t)/X0_og)/dt1/1, d(I(t)/I0)/dt/1, d(Xe(t)/X0)/dt/1, drho_poison/1, To Workspace/1
  Integrator2/1 -> Mux/4
  drho_poison/1 -> Unit Delay/1
  d(Xe(t)/X0)/dt/1 -> Integrator1/1
  Integrator30/1 -> Mux/2
  d(Xe_og(t)/X0_og)/dt1/1 -> Integrator2/1
  d(I(t)/I0)/dt/1 -> Integrator30/1
  drho_Sm_core/1 -> Unit Delay3/1
  Unit Delay3/1 -> Mux1/7, Add/1
  Unit Delay1/1 -> Mux1/3
  FlowFrac/1 -> Mux1/2
  Unit Delay2/1 -> Mux1/6
  d(Sm(t))/dt/1 -> Integrator4/1
  Integrator3/1 -> Mux1/4
  d(Sm_core(t))/dt/1 -> Unit Delay2/1
  Mux1/1 -> To Workspace1/1, d(Pm(t))/dt/1, tau_c(t)/1, d(Sm(t))/dt/1, d(Sm_core(t))/dt/1, drho_Sm_core/1
  Integrator4/1 -> Mux1/5
  n0/1 -> Mux1/1, Mux/1
  d(Pm(t))/dt/1 -> Integrator3/1
  tau_c(t)/1 -> Unit Delay1/1
  Unit Delay/1 -> Add/2, Mux/5
  Add/1 -> drho_Poisson/1

== system MSDR_DH_DeplV1sim/HEAT EXCHANGERS/FUEL FLOW ==
  delay1 : Inport
  delay2 : Inport  Port=2
  delay3 : Inport  Port=3
  Fcn : Fcn  Expr=u[1]/3 + u[2]/3 + u[3]/3
  Mux : Mux
  Tf_out : Outport
  wires:
  delay1/1 -> Mux/1
  delay2/1 -> Mux/2
  delay3/1 -> Mux/3
  Fcn/1 -> Mux/4, Tf_out/1
  Mux/1 -> Fcn/1

== system MSDR_DH_DeplV1sim/HEAT EXCHANGERS/FUEL PUMP 1 ==
  Clock1 : Clock
  Fcn1 : Fcn  Expr=(1-therm_conv)*exp(-K_pump*(u))+therm_conv
  H.T.C. as f(flow_fraction) : Fcn  Expr=0.8215*u^6-4.108*u^5+7.848*u^4-7.165*u^3+3.004*u^2+0.5903*u+0.008537
  Pump Trip Time : TransportDelay  DelayTime=Trip_P1_pump  BufferSize=4096
  FLOW FRACTION : Outport
  HEAT TRANSFER FRACTION : Outport  Port=2
  wires:
  H.T.C. as f(flow_fraction)/1 -> HEAT TRANSFER FRACTION/1
  Clock1/1 -> Pump Trip Time/1
  Pump Trip Time/1 -> Fcn1/1
  Fcn1/1 -> FLOW FRACTION/1, H.T.C. as f(flow_fraction)/1

== system MSDR_DH_DeplV1sim/HEAT EXCHANGERS/FUEL PUMP 2 ==
  Clock1 : Clock
  Fcn1 : Fcn  Expr=(1-therm_conv)*exp(-K_pump*(u))+therm_conv
  H.T.C. as f(flow_fraction) : Fcn  Expr=0.8215*u^6-4.108*u^5+7.848*u^4-7.165*u^3+3.004*u^2+0.5903*u+0.008537
  Pump Trip Time : TransportDelay  DelayTime=Trip_P2_pump  BufferSize=4096
  FLOW FRACTION : Outport
  HEAT TRANSFER FRACTION : Outport  Port=2
  wires:
  Clock1/1 -> Pump Trip Time/1
  H.T.C. as f(flow_fraction)/1 -> HEAT TRANSFER FRACTION/1
  Pump Trip Time/1 -> Fcn1/1
  Fcn1/1 -> FLOW FRACTION/1, H.T.C. as f(flow_fraction)/1

== system MSDR_DH_DeplV1sim/HEAT EXCHANGERS/FUEL PUMP 3 ==
  Clock1 : Clock
  Fcn1 : Fcn  Expr=(1-therm_conv)*exp(-K_pump*(u))+therm_conv
  H.T.C. as f(flow_fraction) : Fcn  Expr=0.8215*u^6-4.108*u^5+7.848*u^4-7.165*u^3+3.004*u^2+0.5903*u+0.008537
  Pump Trip Time : TransportDelay  DelayTime=Trip_P3_pump  BufferSize=4096
  FLOW FRACTION : Outport
  HEAT TRANSFER FRACTION : Outport  Port=2
  wires:
  Fcn1/1 -> FLOW FRACTION/1, H.T.C. as f(flow_fraction)/1
  Clock1/1 -> Pump Trip Time/1
  Pump Trip Time/1 -> Fcn1/1
  H.T.C. as f(flow_fraction)/1 -> HEAT TRANSFER FRACTION/1

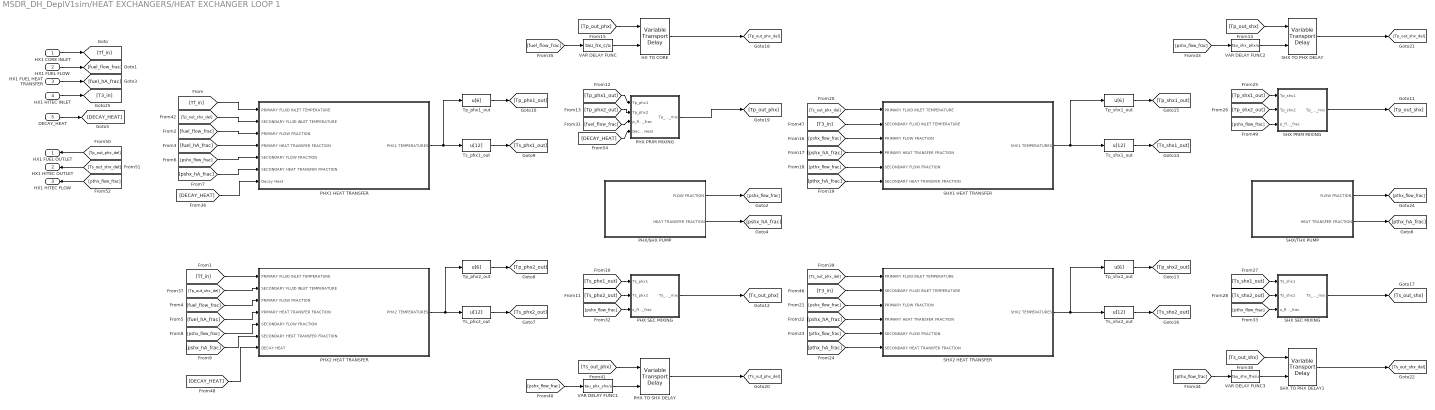
== system MSDR_DH_DeplV1sim/HEAT EXCHANGERS/HEAT EXCHANGER LOOP 1 ==
  HX1 CORE INLET : Inport
  HX1 FUEL FLOW : Inport  Port=2
  HX1 FUEL HEAT TRANSFER : Inport  Port=3
  HX1 HITEC INLET : Inport  Port=4
  DECAY_HEAT : Inport  Port=5
  HX TO CORE : VariableTransportDelay  MaximumDelay=1000000000000  InitialOutput=T0_p_phx1(4)
  PHX PRIM MIXING : Subsystem
  PHX SEC MIXING : Subsystem
  PHX TO SHX DELAY : VariableTransportDelay  MaximumDelay=100000000000  InitialOutput=T0_s_phx1(4)
  PHX/SHX PUMP : Subsystem
  PHX1 HEAT TRANSFER : Subsystem
  PHX2 HEAT TRANSFER : Subsystem
  SHX PRIM MIXING : Subsystem
  SHX SEC MIXING : Subsystem
  SHX TO PHX DELAY : VariableTransportDelay  MaximumDelay=1000000000000  InitialOutput=T0_p_shx1(4)
  SHX TO PHX DELAY1 : VariableTransportDelay  MaximumDelay=1000000000000  InitialOutput=T0_s_shx1(4)
  SHX/THX PUMP : Subsystem
  SHX1 HEAT TRANSFER : Subsystem
  SHX2 HEAT TRANSFER : Subsystem
  Tp_phx1_out : Fcn  Expr=u[6]
  Tp_phx2_out : Fcn  Expr=u[6]
  Tp_shx1_out : Fcn  Expr=u[6]
  Tp_shx2_out : Fcn  Expr=u[6]
  Ts_phx1_out : Fcn  Expr=u[12]
  Ts_phx2_out : Fcn  Expr=u[12]
  Ts_shx1_out : Fcn  Expr=u[12]
  Ts_shx2_out : Fcn  Expr=u[12]
  VAR DELAY FUNC : Fcn  Expr=tau_hx_c/u
  VAR DELAY FUNC1 : Fcn  Expr=tau_phx_shx/u
  VAR DELAY FUNC2 : Fcn  Expr=tau_shx_phx/u
  VAR DELAY FUNC3 : Fcn  Expr=tau_shx_thx/u
  HX1 FUEL OUTLET : Outport
  HX1 HITEC OUTLET : Outport  Port=2
  HX1 HITEC FLOW : Outport  Port=3
  wires:
  PHX1 HEAT TRANSFER/1(PHX1 TEMPERATURES) -> Tp_phx1_out/1, Ts_phx1_out/1
  SHX1 HEAT TRANSFER/1(SHX1 TEMPERATURES) -> Ts_shx1_out/1, Tp_shx1_out/1
  PHX2 HEAT TRANSFER/1(PHX2 TEMPERATURES) -> Tp_phx2_out/1, Ts_phx2_out/1
  SHX2 HEAT TRANSFER/1(SHX2 TEMPERATURES) -> Ts_shx2_out/1, Tp_shx2_out/1
  HX1 CORE INLET/1 -> [Tf_in]
  [Tf_in] -> PHX1 HEAT TRANSFER/1(PRIMARY FLUID INLET TEMPERATURE)
  [Tf_in] -> PHX2 HEAT TRANSFER/1(PRIMARY FLUID INLET TEMPERATURE)
  HX1 FUEL FLOW/1 -> [fuel_flow_frac]
  HX1 FUEL HEAT TRANSFER/1 -> [fuel_hA_frac]
  [fuel_flow_frac] -> PHX1 HEAT TRANSFER/3(PRIMARY FLOW FRACTION)
  [fuel_hA_frac] -> PHX1 HEAT TRANSFER/4(PRIMARY HEAT TRANSFER FRACTION)
  [fuel_flow_frac] -> PHX2 HEAT TRANSFER/3(PRIMARY FLOW FRACTION)
  [fuel_hA_frac] -> PHX2 HEAT TRANSFER/4(PRIMARY HEAT TRANSFER FRACTION)
  PHX/SHX PUMP/2(HEAT TRANSFER FRACTION) -> [pshx_hA_frac]
  PHX/SHX PUMP/1(FLOW FRACTION) -> [pshx_flow_frac]
  SHX/THX PUMP/1(FLOW FRACTION) -> [pthx_flow_frac]
  SHX/THX PUMP/2(HEAT TRANSFER FRACTION) -> [pthx_hA_frac]
  Ts_phx2_out/1 -> [Ts_phx2_out]
  Tp_phx2_out/1 -> [Tp_phx2_out]
  Tp_phx1_out/1 -> [Tp_phx1_out]
  Ts_phx1_out/1 -> [Ts_phx1_out]
  [pshx_flow_frac] -> PHX1 HEAT TRANSFER/5(SECONDARY FLOW FRACTION)
  [pshx_hA_frac] -> PHX1 HEAT TRANSFER/6(SECONDARY HEAT TRANSFER FRACTION)
  [pshx_flow_frac] -> PHX2 HEAT TRANSFER/5(SECONDARY FLOW FRACTION)
  [pshx_hA_frac] -> PHX2 HEAT TRANSFER/6(SECONDARY HEAT TRANSFER FRACTION)
  [Tp_phx1_out] -> PHX PRIM MIXING/1(Tp_phx1)
  [Tp_phx2_out] -> PHX PRIM MIXING/2(Tp_phx2)
  PHX PRIM MIXING/1(Tp_phx_mix) -> [Tp_out_phx]
  [Ts_out_phx_del] -> SHX1 HEAT TRANSFER/1(PRIMARY FLUID INLET TEMPERATURE)
  [pshx_flow_frac] -> SHX1 HEAT TRANSFER/3(PRIMARY FLOW FRACTION)
  [pshx_hA_frac] -> SHX1 HEAT TRANSFER/4(PRIMARY HEAT TRANSFER FRACTION)
  [pthx_flow_frac] -> SHX1 HEAT TRANSFER/5(SECONDARY FLOW FRACTION)
  [pthx_hA_frac] -> SHX1 HEAT TRANSFER/6(SECONDARY HEAT TRANSFER FRACTION)
  [Ts_out_phx_del] -> SHX2 HEAT TRANSFER/1(PRIMARY FLUID INLET TEMPERATURE)
  [pshx_flow_frac] -> SHX2 HEAT TRANSFER/3(PRIMARY FLOW FRACTION)
  [pshx_hA_frac] -> SHX2 HEAT TRANSFER/4(PRIMARY HEAT TRANSFER FRACTION)
  [pthx_flow_frac] -> SHX2 HEAT TRANSFER/5(SECONDARY FLOW FRACTION)
  [pthx_hA_frac] -> SHX2 HEAT TRANSFER/6(SECONDARY HEAT TRANSFER FRACTION)
  Tp_shx1_out/1 -> [Tp_shx1_out]
  Tp_shx2_out/1 -> [Tp_shx2_out]
  Ts_shx1_out/1 -> [Ts_shx1_out]
  Ts_shx2_out/1 -> [Ts_shx2_out]
  [fuel_flow_frac] -> PHX PRIM MIXING/3(p_flow_frac)
  [pshx_flow_frac] -> PHX SEC MIXING/3(s_flow_frac)
  [Ts_phx2_out] -> PHX SEC MIXING/2(Ts_phx2)
  [Ts_phx1_out] -> PHX SEC MIXING/1(Ts_phx1)
  PHX SEC MIXING/1(Ts_phx_mix) -> [Ts_out_phx]
  [Tp_shx2_out] -> SHX PRIM MIXING/2(Tp_shx2)
  [Tp_shx1_out] -> SHX PRIM MIXING/1(Tp_shx1)
  SHX PRIM MIXING/1(Tp_shx_mix) -> [Tp_out_shx]
  [Ts_shx1_out] -> SHX SEC MIXING/1(Ts_shx1)
  SHX SEC MIXING/1(Ts_shx_mix) -> [Ts_out_shx]
  [Ts_shx2_out] -> SHX SEC MIXING/2(Ts_shx2)
  [pthx_flow_frac] -> SHX SEC MIXING/3(s_flow_frac)
  [Tp_out_shx_del] -> PHX1 HEAT TRANSFER/2(SECONDARY FLUID INLET TEMPERATURE)
  [Tp_out_shx_del] -> PHX2 HEAT TRANSFER/2(SECONDARY FLUID INLET TEMPERATURE)
  VAR DELAY FUNC/1 -> HX TO CORE/2
  [Tp_out_phx] -> HX TO CORE/1
  [fuel_flow_frac] -> VAR DELAY FUNC/1
  HX TO CORE/1 -> [Tp_out_phx_del]
  VAR DELAY FUNC1/1 -> PHX TO SHX DELAY/2
  PHX TO SHX DELAY/1 -> [Ts_out_phx_del]
  [Ts_out_phx] -> PHX TO SHX DELAY/1
  [pshx_flow_frac] -> VAR DELAY FUNC1/1
  VAR DELAY FUNC2/1 -> SHX TO PHX DELAY/2
  SHX TO PHX DELAY/1 -> [Tp_out_shx_del]
  [pshx_flow_frac] -> VAR DELAY FUNC2/1
  [Tp_out_shx] -> SHX TO PHX DELAY/1
  [Ts_out_shx] -> SHX TO PHX DELAY1/1
  [pthx_flow_frac] -> VAR DELAY FUNC3/1
  SHX TO PHX DELAY1/1 -> [Ts_out_shx_del]
  VAR DELAY FUNC3/1 -> SHX TO PHX DELAY1/2
  [T3_in] -> SHX1 HEAT TRANSFER/2(SECONDARY FLUID INLET TEMPERATURE)
  [T3_in] -> SHX2 HEAT TRANSFER/2(SECONDARY FLUID INLET TEMPERATURE)
  HX1 HITEC INLET/1 -> [T3_in]
  [pshx_flow_frac] -> SHX PRIM MIXING/3(p_flow_frac)
  [pthx_flow_frac] -> HX1 HITEC FLOW/1
  [Ts_out_shx_del] -> HX1 HITEC OUTLET/1
  [Tp_out_phx_del] -> HX1 FUEL OUTLET/1
  DECAY_HEAT/1 -> [DECAY_HEAT]
  [DECAY_HEAT] -> PHX1 HEAT TRANSFER/7(Decay Heat)
  [DECAY_HEAT] -> PHX2 HEAT TRANSFER/7(DECAY HEAT)
  [DECAY_HEAT] -> PHX PRIM MIXING/4(Decay Heat)

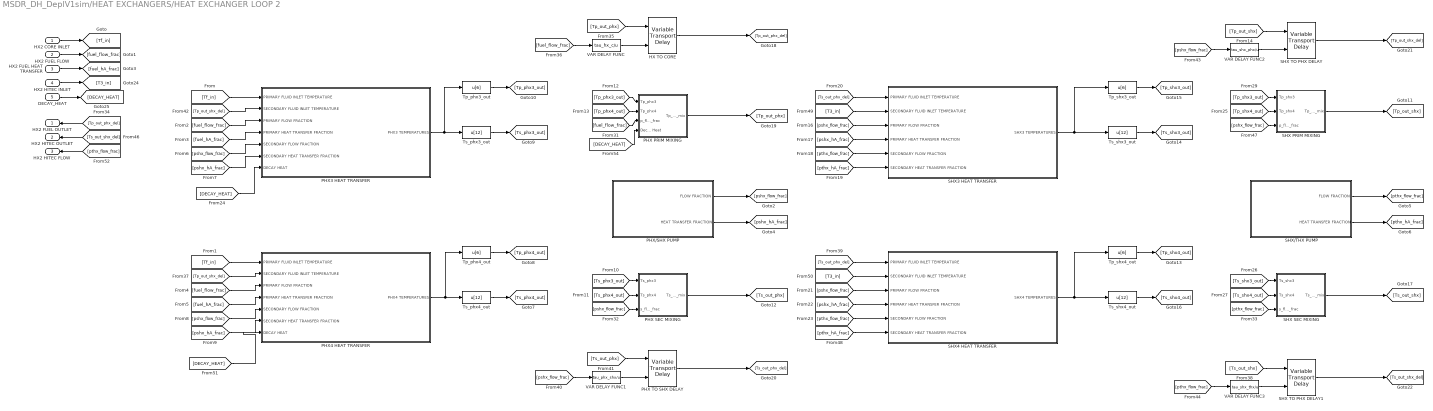
== system MSDR_DH_DeplV1sim/HEAT EXCHANGERS/HEAT EXCHANGER LOOP 2 ==
  HX2 CORE INLET : Inport
  HX2 FUEL FLOW : Inport  Port=2
  HX2 FUEL HEAT TRANSFER : Inport  Port=3
  HX2 HITEC INLET : Inport  Port=4
  DECAY_HEAT : Inport  Port=5
  HX TO CORE : VariableTransportDelay  MaximumDelay=1000000000000  InitialOutput=T0_p_phx3(4)
  PHX PRIM MIXING : Subsystem
  PHX SEC MIXING : Subsystem
  PHX TO SHX DELAY : VariableTransportDelay  MaximumDelay=100000000000  InitialOutput=T0_s_phx3(4)
  PHX/SHX PUMP : Subsystem
  PHX3 HEAT TRANSFER : Subsystem
  PHX4 HEAT TRANSFER : Subsystem
  SHX PRIM MIXING : Subsystem
  SHX SEC MIXING : Subsystem
  SHX TO PHX DELAY : VariableTransportDelay  MaximumDelay=1000000000000  InitialOutput=T0_p_shx3(4)
  SHX TO PHX DELAY1 : VariableTransportDelay  MaximumDelay=1000000000000  InitialOutput=T0_s_shx3(4)
  SHX/THX PUMP : Subsystem
  SHX3 HEAT TRANSFER : Subsystem
  SHX4 HEAT TRANSFER : Subsystem
  Tp_phx3_out : Fcn  Expr=u[6]
  Tp_phx4_out : Fcn  Expr=u[6]
  Tp_shx3_out : Fcn  Expr=u[6]
  Tp_shx4_out : Fcn  Expr=u[6]
  Ts_phx3_out : Fcn  Expr=u[12]
  Ts_phx4_out : Fcn  Expr=u[12]
  Ts_shx3_out : Fcn  Expr=u[12]
  Ts_shx4_out : Fcn  Expr=u[12]
  VAR DELAY FUNC : Fcn  Expr=tau_hx_c/u
  VAR DELAY FUNC1 : Fcn  Expr=tau_phx_shx/u
  VAR DELAY FUNC2 : Fcn  Expr=tau_shx_phx/u
  VAR DELAY FUNC3 : Fcn  Expr=tau_shx_thx/u
  HX2 FUEL OUTLET : Outport
  HX2 HITEC OUTLET : Outport  Port=2
  HX2 HITEC FLOW : Outport  Port=3
  wires:
  [Tp_out_phx_del] -> HX2 FUEL OUTLET/1
  HX2 CORE INLET/1 -> [Tf_in]
  HX2 FUEL HEAT TRANSFER/1 -> [fuel_hA_frac]
  HX2 FUEL FLOW/1 -> [fuel_flow_frac]
  Tp_phx3_out/1 -> [Tp_phx3_out]
  PHX3 HEAT TRANSFER/1(PHX3 TEMPERATURES) -> Tp_phx3_out/1, Ts_phx3_out/1
  Ts_phx3_out/1 -> [Ts_phx3_out]
  Tp_phx4_out/1 -> [Tp_phx4_out]
  Ts_phx4_out/1 -> [Ts_phx4_out]
  PHX4 HEAT TRANSFER/1(PHX4 TEMPERATURES) -> Tp_phx4_out/1, Ts_phx4_out/1
  Tp_shx3_out/1 -> [Tp_shx3_out]
  Ts_shx3_out/1 -> [Ts_shx3_out]
  SHX3 HEAT TRANSFER/1(SHX3 TEMPERATURES) -> Ts_shx3_out/1, Tp_shx3_out/1
  [Tp_phx3_out] -> PHX PRIM MIXING/1(Tp_phx3)
  [fuel_flow_frac] -> PHX PRIM MIXING/3(p_flow_frac)
  [Ts_phx3_out] -> PHX SEC MIXING/1(Ts_phx3)
  [Ts_phx4_out] -> PHX SEC MIXING/2(Ts_phx4)
  [Tp_phx4_out] -> PHX PRIM MIXING/2(Tp_phx4)
  PHX SEC MIXING/1(Ts_phx_mix) -> [Ts_out_phx]
  PHX/SHX PUMP/1(FLOW FRACTION) -> [pshx_flow_frac]
  PHX PRIM MIXING/1(Tp_phx_mix) -> [Tp_out_phx]
  [pshx_flow_frac] -> PHX SEC MIXING/3(s_flow_frac)
  PHX/SHX PUMP/2(HEAT TRANSFER FRACTION) -> [pshx_hA_frac]
  Tp_shx4_out/1 -> [Tp_shx4_out]
  SHX4 HEAT TRANSFER/1(SHX4 TEMPERATURES) -> Ts_shx4_out/1, Tp_shx4_out/1
  Ts_shx4_out/1 -> [Ts_shx4_out]
  [Tp_shx3_out] -> SHX PRIM MIXING/1(Tp_shx3)
  [Ts_shx4_out] -> SHX SEC MIXING/2(Ts_shx4)
  [Ts_shx3_out] -> SHX SEC MIXING/1(Ts_shx3)
  [Tp_shx4_out] -> SHX PRIM MIXING/2(Tp_shx4)
  SHX/THX PUMP/2(HEAT TRANSFER FRACTION) -> [pthx_hA_frac]
  SHX SEC MIXING/1(Ts_shx_mix) -> [Ts_out_shx]
  SHX PRIM MIXING/1(Tp_shx_mix) -> [Tp_out_shx]
  SHX/THX PUMP/1(FLOW FRACTION) -> [pthx_flow_frac]
  [pthx_flow_frac] -> SHX SEC MIXING/3(s_flow_frac)
  [fuel_hA_frac] -> PHX3 HEAT TRANSFER/4(PRIMARY HEAT TRANSFER FRACTION)
  [Tp_out_shx_del] -> PHX3 HEAT TRANSFER/2(SECONDARY FLUID INLET TEMPERATURE)
  [pshx_hA_frac] -> PHX3 HEAT TRANSFER/6(SECONDARY HEAT TRANSFER FRACTION)
  [Tf_in] -> PHX3 HEAT TRANSFER/1(PRIMARY FLUID INLET TEMPERATURE)
  [pshx_flow_frac] -> PHX3 HEAT TRANSFER/5(SECONDARY FLOW FRACTION)
  [fuel_flow_frac] -> PHX3 HEAT TRANSFER/3(PRIMARY FLOW FRACTION)
  [Tp_out_shx_del] -> PHX4 HEAT TRANSFER/2(SECONDARY FLUID INLET TEMPERATURE)
  [pshx_flow_frac] -> PHX4 HEAT TRANSFER/5(SECONDARY FLOW FRACTION)
  [fuel_flow_frac] -> PHX4 HEAT TRANSFER/3(PRIMARY FLOW FRACTION)
  [Tf_in] -> PHX4 HEAT TRANSFER/1(PRIMARY FLUID INLET TEMPERATURE)
  [pshx_hA_frac] -> PHX4 HEAT TRANSFER/6(SECONDARY HEAT TRANSFER FRACTION)
  [fuel_hA_frac] -> PHX4 HEAT TRANSFER/4(PRIMARY HEAT TRANSFER FRACTION)
  VAR DELAY FUNC/1 -> HX TO CORE/2
  HX TO CORE/1 -> [Tp_out_phx_del]
  [Tp_out_phx] -> HX TO CORE/1
  [fuel_flow_frac] -> VAR DELAY FUNC/1
  [Ts_out_phx] -> PHX TO SHX DELAY/1
  [pshx_flow_frac] -> VAR DELAY FUNC1/1
  VAR DELAY FUNC1/1 -> PHX TO SHX DELAY/2
  PHX TO SHX DELAY/1 -> [Ts_out_phx_del]
  [pthx_flow_frac] -> SHX3 HEAT TRANSFER/5(SECONDARY FLOW FRACTION)
  [pthx_hA_frac] -> SHX3 HEAT TRANSFER/6(SECONDARY HEAT TRANSFER FRACTION)
  [pshx_hA_frac] -> SHX3 HEAT TRANSFER/4(PRIMARY HEAT TRANSFER FRACTION)
  [Ts_out_phx_del] -> SHX3 HEAT TRANSFER/1(PRIMARY FLUID INLET TEMPERATURE)
  [pshx_flow_frac] -> SHX3 HEAT TRANSFER/3(PRIMARY FLOW FRACTION)
  [pthx_hA_frac] -> SHX4 HEAT TRANSFER/6(SECONDARY HEAT TRANSFER FRACTION)
  [pthx_flow_frac] -> SHX4 HEAT TRANSFER/5(SECONDARY FLOW FRACTION)
  [pshx_hA_frac] -> SHX4 HEAT TRANSFER/4(PRIMARY HEAT TRANSFER FRACTION)
  [pshx_flow_frac] -> SHX4 HEAT TRANSFER/3(PRIMARY FLOW FRACTION)
  [Ts_out_phx_del] -> SHX4 HEAT TRANSFER/1(PRIMARY FLUID INLET TEMPERATURE)
  [Tp_out_shx] -> SHX TO PHX DELAY/1
  [pshx_flow_frac] -> VAR DELAY FUNC2/1
  SHX TO PHX DELAY/1 -> [Tp_out_shx_del]
  VAR DELAY FUNC2/1 -> SHX TO PHX DELAY/2
  VAR DELAY FUNC3/1 -> SHX TO PHX DELAY1/2
  SHX TO PHX DELAY1/1 -> [Ts_out_shx_del]
  [Ts_out_shx] -> SHX TO PHX DELAY1/1
  [pthx_flow_frac] -> VAR DELAY FUNC3/1
  [T3_in] -> SHX3 HEAT TRANSFER/2(SECONDARY FLUID INLET TEMPERATURE)
  [T3_in] -> SHX4 HEAT TRANSFER/2(SECONDARY FLUID INLET TEMPERATURE)
  HX2 HITEC INLET/1 -> [T3_in]
  [Ts_out_shx_del] -> HX2 HITEC OUTLET/1
  [pshx_flow_frac] -> SHX PRIM MIXING/3(p_flow_frac)
  [pthx_flow_frac] -> HX2 HITEC FLOW/1
  DECAY_HEAT/1 -> [DECAY_HEAT]
  [DECAY_HEAT] -> PHX3 HEAT TRANSFER/7(DECAY HEAT)
  [DECAY_HEAT] -> PHX4 HEAT TRANSFER/7(DECAY HEAT)
  [DECAY_HEAT] -> PHX PRIM MIXING/4(Decay Heat)

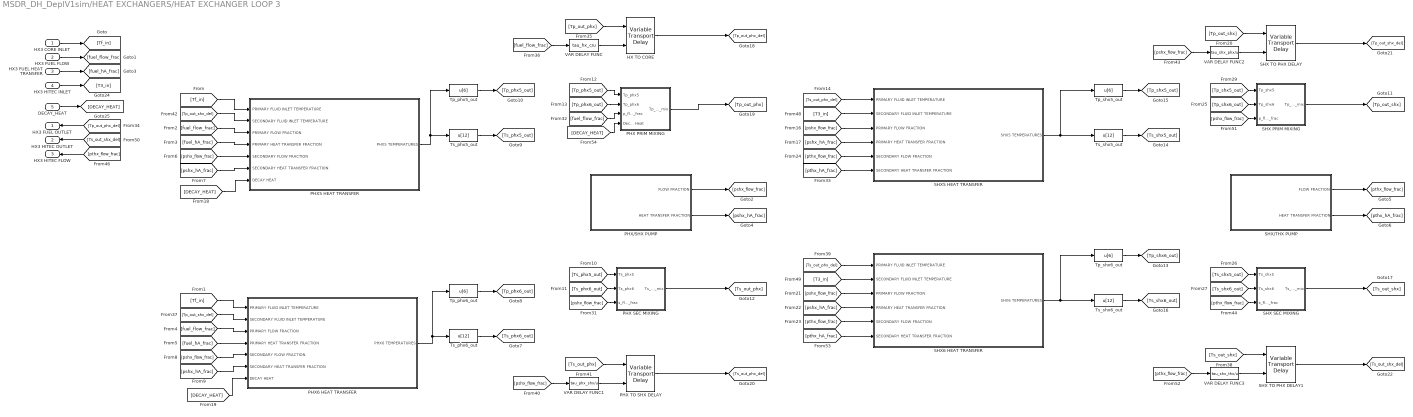
== system MSDR_DH_DeplV1sim/HEAT EXCHANGERS/HEAT EXCHANGER LOOP 3 ==
  HX3 CORE INLET : Inport
  HX3 FUEL FLOW : Inport  Port=2
  HX3 FUEL HEAT TRANSFER : Inport  Port=3
  HX3 HITEC INLET : Inport  Port=4
  DECAY_HEAT : Inport  Port=5
  HX TO CORE : VariableTransportDelay  MaximumDelay=1000000000000  InitialOutput=T0_p_phx5(4)
  PHX PRIM MIXING : Subsystem
  PHX SEC MIXING : Subsystem
  PHX TO SHX DELAY : VariableTransportDelay  MaximumDelay=100000000000  InitialOutput=T0_s_phx5(4)
  PHX/SHX PUMP : Subsystem
  PHX5 HEAT TRANSFER : Subsystem
  PHX6 HEAT TRANSFER : Subsystem
  SHX PRIM MIXING : Subsystem
  SHX SEC MIXING : Subsystem
  SHX TO PHX DELAY : VariableTransportDelay  MaximumDelay=1000000000000  InitialOutput=T0_p_shx5(4)
  SHX TO PHX DELAY1 : VariableTransportDelay  MaximumDelay=1000000000000  InitialOutput=T0_s_shx5(4)
  SHX/THX PUMP : Subsystem
  SHX5 HEAT TRANSFER : Subsystem
  SHX6 HEAT TRANSFER : Subsystem
  Tp_phx5_out : Fcn  Expr=u[6]
  Tp_phx6_out : Fcn  Expr=u[6]
  Tp_shx5_out : Fcn  Expr=u[6]
  Tp_shx6_out : Fcn  Expr=u[6]
  Ts_phx5_out : Fcn  Expr=u[12]
  Ts_phx6_out : Fcn  Expr=u[12]
  Ts_shx5_out : Fcn  Expr=u[12]
  Ts_shx6_out : Fcn  Expr=u[12]
  VAR DELAY FUNC : Fcn  Expr=tau_hx_c/u
  VAR DELAY FUNC1 : Fcn  Expr=tau_phx_shx/u
  VAR DELAY FUNC2 : Fcn  Expr=tau_shx_phx/u
  VAR DELAY FUNC3 : Fcn  Expr=tau_shx_thx/u
  HX3 FUEL OUTLET : Outport
  HX3 HITEC OUTLET : Outport  Port=2
  HX3 HITEC FLOW : Outport  Port=3
  wires:
  HX3 FUEL FLOW/1 -> [fuel_flow_frac]
  HX3 FUEL HEAT TRANSFER/1 -> [fuel_hA_frac]
  HX3 CORE INLET/1 -> [Tf_in]
  [Tp_out_phx_del] -> HX3 FUEL OUTLET/1
  PHX5 HEAT TRANSFER/1(PHX5 TEMPERATURES) -> Tp_phx5_out/1, Ts_phx5_out/1
  Tp_phx5_out/1 -> [Tp_phx5_out]
  Ts_phx5_out/1 -> [Ts_phx5_out]
  PHX6 HEAT TRANSFER/1(PHX6 TEMPERATURES) -> Tp_phx6_out/1, Ts_phx6_out/1
  Tp_phx6_out/1 -> [Tp_phx6_out]
  Ts_phx6_out/1 -> [Ts_phx6_out]
  PHX/SHX PUMP/2(HEAT TRANSFER FRACTION) -> [pshx_hA_frac]
  [pshx_flow_frac] -> PHX SEC MIXING/3(s_flow_frac)
  [Ts_phx5_out] -> PHX SEC MIXING/1(Ts_phx5)
  PHX/SHX PUMP/1(FLOW FRACTION) -> [pshx_flow_frac]
  [Ts_phx6_out] -> PHX SEC MIXING/2(Ts_phx6)
  PHX SEC MIXING/1(Ts_phx_mix) -> [Ts_out_phx]
  [Tp_phx6_out] -> PHX PRIM MIXING/2(Tp_phx6)
  PHX PRIM MIXING/1(Tp_phx_mix) -> [Tp_out_phx]
  [Tp_phx5_out] -> PHX PRIM MIXING/1(Tp_phx5)
  [fuel_flow_frac] -> PHX PRIM MIXING/3(p_flow_frac)
  Ts_shx5_out/1 -> [Ts_shx5_out]
  Tp_shx5_out/1 -> [Tp_shx5_out]
  SHX5 HEAT TRANSFER/1(SHX5 TEMPERATURES) -> Ts_shx5_out/1, Tp_shx5_out/1
  SHX6 HEAT TRANSFER/1(SHX6 TEMPERATURES) -> Ts_shx6_out/1, Tp_shx6_out/1
  Ts_shx6_out/1 -> [Ts_shx6_out]
  Tp_shx6_out/1 -> [Tp_shx6_out]
  SHX/THX PUMP/1(FLOW FRACTION) -> [pthx_flow_frac]
  SHX SEC MIXING/1(Ts_shx_mix) -> [Ts_out_shx]
  SHX/THX PUMP/2(HEAT TRANSFER FRACTION) -> [pthx_hA_frac]
  SHX PRIM MIXING/1(Tp_shx_mix) -> [Tp_out_shx]
  [Ts_shx5_out] -> SHX SEC MIXING/1(Ts_shx5)
  [Tp_shx5_out] -> SHX PRIM MIXING/1(Tp_shx5)
  [pthx_flow_frac] -> SHX SEC MIXING/3(s_flow_frac)
  [Ts_shx6_out] -> SHX SEC MIXING/2(Ts_shx6)
  [Tp_shx6_out] -> SHX PRIM MIXING/2(Tp_shx6)
  [pshx_hA_frac] -> PHX5 HEAT TRANSFER/6(SECONDARY HEAT TRANSFER FRACTION)
  [Tp_out_shx_del] -> PHX5 HEAT TRANSFER/2(SECONDARY FLUID INLET TEMPERATURE)
  [pshx_flow_frac] -> PHX5 HEAT TRANSFER/5(SECONDARY FLOW FRACTION)
  [fuel_hA_frac] -> PHX5 HEAT TRANSFER/4(PRIMARY HEAT TRANSFER FRACTION)
  [Tf_in] -> PHX5 HEAT TRANSFER/1(PRIMARY FLUID INLET TEMPERATURE)
  [fuel_flow_frac] -> PHX5 HEAT TRANSFER/3(PRIMARY FLOW FRACTION)
  [pshx_flow_frac] -> PHX6 HEAT TRANSFER/5(SECONDARY FLOW FRACTION)
  [fuel_hA_frac] -> PHX6 HEAT TRANSFER/4(PRIMARY HEAT TRANSFER FRACTION)
  [pshx_hA_frac] -> PHX6 HEAT TRANSFER/6(SECONDARY HEAT TRANSFER FRACTION)
  [Tf_in] -> PHX6 HEAT TRANSFER/1(PRIMARY FLUID INLET TEMPERATURE)
  [fuel_flow_frac] -> PHX6 HEAT TRANSFER/3(PRIMARY FLOW FRACTION)
  [Tp_out_shx_del] -> PHX6 HEAT TRANSFER/2(SECONDARY FLUID INLET TEMPERATURE)
  [fuel_flow_frac] -> VAR DELAY FUNC/1
  [Tp_out_phx] -> HX TO CORE/1
  HX TO CORE/1 -> [Tp_out_phx_del]
  VAR DELAY FUNC/1 -> HX TO CORE/2
  PHX TO SHX DELAY/1 -> [Ts_out_phx_del]
  [pshx_flow_frac] -> VAR DELAY FUNC1/1
  VAR DELAY FUNC1/1 -> PHX TO SHX DELAY/2
  [Ts_out_phx] -> PHX TO SHX DELAY/1
  [pshx_flow_frac] -> SHX5 HEAT TRANSFER/3(PRIMARY FLOW FRACTION)
  [pshx_hA_frac] -> SHX5 HEAT TRANSFER/4(PRIMARY HEAT TRANSFER FRACTION)
  [pthx_hA_frac] -> SHX5 HEAT TRANSFER/6(SECONDARY HEAT TRANSFER FRACTION)
  [Ts_out_phx_del] -> SHX5 HEAT TRANSFER/1(PRIMARY FLUID INLET TEMPERATURE)
  [pthx_flow_frac] -> SHX5 HEAT TRANSFER/5(SECONDARY FLOW FRACTION)
  [pthx_hA_frac] -> SHX6 HEAT TRANSFER/6(SECONDARY HEAT TRANSFER FRACTION)
  [pshx_hA_frac] -> SHX6 HEAT TRANSFER/4(PRIMARY HEAT TRANSFER FRACTION)
  [pshx_flow_frac] -> SHX6 HEAT TRANSFER/3(PRIMARY FLOW FRACTION)
  [pthx_flow_frac] -> SHX6 HEAT TRANSFER/5(SECONDARY FLOW FRACTION)
  [Ts_out_phx_del] -> SHX6 HEAT TRANSFER/1(PRIMARY FLUID INLET TEMPERATURE)
  VAR DELAY FUNC2/1 -> SHX TO PHX DELAY/2
  [Tp_out_shx] -> SHX TO PHX DELAY/1
  [pshx_flow_frac] -> VAR DELAY FUNC2/1
  SHX TO PHX DELAY/1 -> [Tp_out_shx_del]
  [Ts_out_shx] -> SHX TO PHX DELAY1/1
  SHX TO PHX DELAY1/1 -> [Ts_out_shx_del]
  [pthx_flow_frac] -> VAR DELAY FUNC3/1
  VAR DELAY FUNC3/1 -> SHX TO PHX DELAY1/2
  [T3_in] -> SHX5 HEAT TRANSFER/2(SECONDARY FLUID INLET TEMPERATURE)
  [T3_in] -> SHX6 HEAT TRANSFER/2(SECONDARY FLUID INLET TEMPERATURE)
  HX3 HITEC INLET/1 -> [T3_in]
  [Ts_out_shx_del] -> HX3 HITEC OUTLET/1
  [pthx_flow_frac] -> HX3 HITEC FLOW/1
  [pshx_flow_frac] -> SHX PRIM MIXING/3(p_flow_frac)
  DECAY_HEAT/1 -> [DECAY_HEAT]
  [DECAY_HEAT] -> PHX5 HEAT TRANSFER/7(DECAY HEAT)
  [DECAY_HEAT] -> PHX6 HEAT TRANSFER/7(DECAY HEAT)
  [DECAY_HEAT] -> PHX PRIM MIXING/4(Decay Heat)

== system MSDR_DH_DeplV1sim/HEAT EXCHANGERS/HITEC FLOW ==
  delay1 : Inport
  delay2 : Inport  Port=2
  delay3 : Inport  Port=3
  Fcn : Fcn  Expr=u[1]/3 + u[2]/3 + u[3]/3
  Mux : Mux
  Tf_out : Outport
  wires:
  delay1/1 -> Mux/1
  delay2/1 -> Mux/2
  delay3/1 -> Mux/3
  Fcn/1 -> Mux/4, Tf_out/1
  Mux/1 -> Fcn/1

== system MSDR_DH_DeplV1sim/HEAT EXCHANGERS/PRE BoP MIXING ==
  Tshx1 : Inport
  delay1 : Inport  Port=2
  Tshx2 : Inport  Port=3
  delay2 : Inport  Port=4
  Tshx3 : Inport  Port=5
  delay3 : Inport  Port=6
  Fcn : Fcn  Expr=u[2]*W_31/m_3m*(u[1] - u[7]) + u[4]*W_32/m_3m*(u[3] - u[7]) + u[6]*W_33/m_3m*(u[5] - u[7])
  Integrator : Integrator  InitialCondition=T3_out
  Mux : Mux  Inputs=7
  T3_out : Outport
  wires:
  Tshx1/1 -> Mux/1
  delay1/1 -> Mux/2
  Tshx2/1 -> Mux/3
  delay2/1 -> Mux/4
  Tshx3/1 -> Mux/5
  delay3/1 -> Mux/6
  Mux/1 -> Fcn/1
  Fcn/1 -> Integrator/1
  Integrator/1 -> T3_out/1, Mux/7

== system MSDR_DH_DeplV1sim/HEAT EXCHANGERS/PRE CORE MIXING ==
  Tphx1 : Inport
  delay1 : Inport  Port=2
  Tphx2 : Inport  Port=3
  delay2 : Inport  Port=4
  Tphx3 : Inport  Port=5
  delay3 : Inport  Port=6
  Decay Heat : Inport  Port=7
  Clock : Clock
  DHRS MODE : Constant  Value=DHRS_MODE
  Display1 : Display
  Display2 : Display
  Fcn : Fcn  Expr=u[2]*W_f1/m_fm*(u[1] - u[7]) + u[4]*W_f2/m_fm*(u[3] - u[7]) + u[6]*W_f3/m_fm*(u[5] - u[7]) - u[10]/(m_fm*Cp_f) + (u[8]*P*m_fm)/(m_f_t*m_fm*Cp_f)
  Integrator : Integrator  InitialCondition=Tf_in
  Mux : Mux  Inputs=10
      settings: DisplayOption=signals
  "NORNAML DHRS " : Fcn  Expr=(DHRS_Power-Power_Bleed)/(1+exp(ln(1/Epsilon - 1)*(1 - (u[9]-DHRS_time)/DHRS_TIME_K)))+Power_Bleed
  SLUG DATA : FromWorkspace  VariableName=slugger  SampleTime=1  Interpolate=off  OutputAfterFinalValue=Holding final value
  Scope : Scope
  Switch : Switch  Threshold=2
  Tf_out : Outport
  wires:
  Tphx1/1 -> Mux/1
  delay1/1 -> Mux/2
  Tphx2/1 -> Mux/3
  delay2/1 -> Mux/4
  Tphx3/1 -> Mux/5
  delay3/1 -> Mux/6
  Mux/1 -> "NORNAML DHRS "/1, Fcn/1
  Fcn/1 -> Integrator/1
  Integrator/1 -> Mux/7, Display1/1, Scope/1, Tf_out/1
  Clock/1 -> Mux/9
  Decay Heat/1 -> Mux/8
  Switch/1 -> Display2/1, Mux/10
  "NORNAML DHRS "/1 -> Switch/3
  SLUG DATA/1 -> Switch/1
  DHRS MODE/1 -> Switch/2
